simulink model "exp06"  (R2018a)
settings: Solver=VariableStepAuto  StartTime=0.0  StopTime=10.0  RelTol=1e-3
libraries: simulink x1
settings Model: Creator=Administrator  LastModifiedBy=Administrator

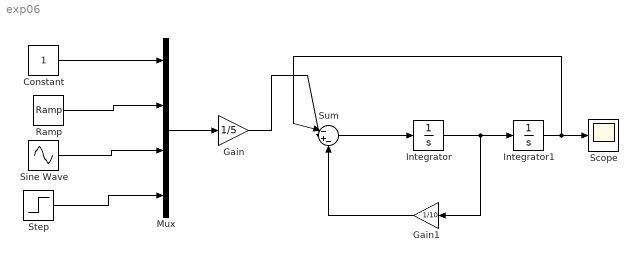
== system exp06 ==
  Constant : Constant
  Gain : Gain  Gain=1/5
  Gain1 : Gain  Gain=1/10
  Integrator : Integrator
  Integrator1 : Integrator
  Mux : Mux
  Ramp : simulink/Sources/Ramp  slope=1  start=0  InitialOutput=0
  Scope : Scope
  Sine Wave : Sin  SampleTime=0
  Step : Step  SampleTime=0
  Sum : Sum  Inputs=|-+-
  wires:
  Constant/1 -> Mux/1
  Ramp/1 -> Mux/2
  Sine Wave/1 -> Mux/3
  Step/1 -> Mux/4
  Mux/1 -> Gain/1
  Gain/1 -> Sum/2
  Integrator1/1 -> Sum/1, Scope/1
  Gain1/1 -> Sum/3
  Sum/1 -> Integrator/1
  Integrator/1 -> Gain1/1, Integrator1/1
